simulink model "CLIK_Jpseudo_inv"  (R2023b)
settings: Solver=ode1  StartTime=0.0  StopTime=50  FixedStep=Tc  RelTol=1e-3
values from neighbouring files (symbols this model uses):
  Tc = 0.001    [scara_parameters.m]
undefined symbols (not defined in the file or in its folder): DiscIntNeverNeededParam, k0, K_Jpseudo_inv, q0
settings Model: Creator=emman  LastModifiedBy=emman

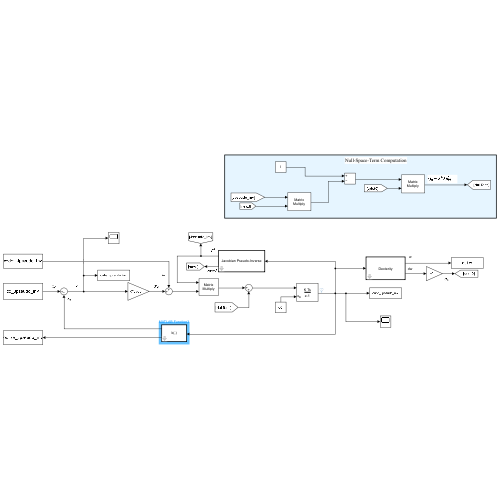
[thumbnail: Simulink's stored preview of the top-level diagram]
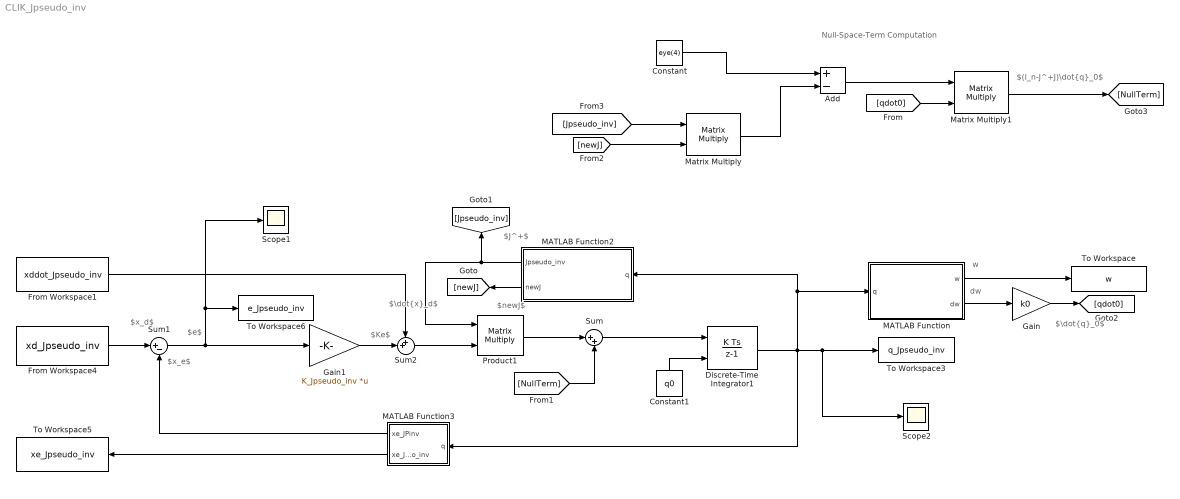
== system CLIK_Jpseudo_inv ==
  note: Null-Space-Term Computation
  note: $(I_n-J^+J)\dot{q}_0$
  note: $newJ$
  note: $J^+$
  note: $\dot{q}_0$
  note: dw
  note: w
  note: $Ke$
  note: $e$
  note: $\dot{x}_d$
  note: $x_d$
  note: $x_e$
  Add : Sum  Inputs=+-
  Constant : Constant  Value=eye(4)
      mask Display: disp('I');
  Constant1 : Constant  Value=q0
  Discrete-Time Integrator1 : DiscreteIntegrator  InitialConditionSource=external  InitialCondition=q0  SampleTime=Tc  ICPrevOutput=DiscIntNeverNeededParam  ICPrevScaledInput=DiscIntNeverNeededParam
  From Workspace1 : FromWorkspace  VariableName=xddot_Jpseudo_inv  SampleTime=Tc
  From Workspace4 : FromWorkspace  VariableName=xd_Jpseudo_inv  SampleTime=Tc
  Gain : Gain  Gain=k0
  Gain1 : Gain  Gain=K_Jpseudo_inv  Multiplication=Matrix(K*u) (u vector)
  MATLAB Function : MATLAB Function  TreatAsAtomicUnit=on
  MATLAB Function2 : MATLAB Function  TreatAsAtomicUnit=on
  MATLAB Function3 : MATLAB Function  TreatAsAtomicUnit=on
  Matrix Multiply : Product  Multiplication=Matrix(*)
  Matrix Multiply1 : Product  Multiplication=Matrix(*)
  Product1 : Product  Multiplication=Matrix(*)
  Scope1 : Scope
  Scope2 : Scope
  Sum : Sum  Inputs=|++
  Sum1 : Sum  Inputs=|+-
  Sum2 : Sum  Inputs=++|
  To Workspace : ToWorkspace  VariableName=w  SaveFormat=Structure With Time  SampleTime=-1
  To Workspace3 : ToWorkspace  VariableName=q_Jpseudo_inv  SaveFormat=Structure With Time  SampleTime=-1
  To Workspace5 : ToWorkspace  VariableName=xe_Jpseudo_inv  SaveFormat=Structure With Time  SampleTime=-1
  To Workspace6 : ToWorkspace  VariableName=e_Jpseudo_inv  SaveFormat=Structure With Time  SampleTime=-1
  wires:
  Discrete-Time Integrator1/1 -> MATLAB Function2/1(q), MATLAB Function/1(q), To Workspace3/1, Scope2/1, MATLAB Function3/1(q)
  From Workspace4/1 -> Sum1/1
  From Workspace1/1 -> Sum2/1
  Constant1/1 -> Discrete-Time Integrator1/2
  MATLAB Function2/1(Jpseudo_inv) -> Product1/1, [Jpseudo_inv]
  Gain1/1 -> Sum2/2
  Sum2/1 -> Product1/2
  Sum1/1 -> Scope1/1, To Workspace6/1, Gain1/1
  MATLAB Function/1(w) -> To Workspace/1
  MATLAB Function/2(dw) -> Gain/1
  MATLAB Function2/2(newJ) -> [newJ]
  Constant/1 -> Add/1
  [Jpseudo_inv] -> Matrix Multiply/1
  [newJ] -> Matrix Multiply/2
  Matrix Multiply/1 -> Add/2
  Gain/1 -> [qdot0]
  Add/1 -> Matrix Multiply1/1
  [qdot0] -> Matrix Multiply1/2
  Matrix Multiply1/1 -> [NullTerm]
  Product1/1 -> Sum/1
  Sum/1 -> Discrete-Time Integrator1/1
  [NullTerm] -> Sum/2
  MATLAB Function3/1(xe_JPinv) -> Sum1/2
  MATLAB Function3/2(xe_JPseudo_inv) -> To Workspace5/1

== matlab function CLIK_Jpseudo_inv/MATLAB Function2 ==
  data: Jpseudo_inv output; q input; newJ output
function [Jpseudo_inv,newJ] = JacobianPseudoInverse(q)

    a1 = 0.5;
    a2 = 0.5;
    
    newJ = [-a2*sin(q(1)+q(2))-a1*sin(q(1)) -a2*sin(q(1)+q(2)) 0 0;
        %a2*cos(q(1)+q(2))+a1*cos(q(1)) a2*cos(q(1)+q(2)) 0 0;
        0 0 -1 0;
        1 1 0 -1];

    Jpseudo_inv = newJ'*inv(newJ*newJ');

end

== matlab function CLIK_Jpseudo_inv/MATLAB Function3 ==
  data: xe_JPinv output; q input; xe_JPseudo_inv output
function [xe_JPinv, xe_JPseudo_inv] = DirKinPseudoInv(q)
    
    a1 = 0.5;
    a2 = 0.5;
    d0 = 1;
    
    xe_JPinv = [a2*cos(q(1)+q(2))+a1*cos(q(1));
       %a2*sin(q(1)+q(2))+a1*sin(q(1));
       d0-q(3);
       q(1)+q(2)-q(4)];

    xe_JPseudo_inv = [a2*cos(q(1)+q(2))+a1*cos(q(1));
       a2*sin(q(1)+q(2))+a1*sin(q(1));
       d0-q(3);
       q(1)+q(2)-q(4)];

end

== matlab function CLIK_Jpseudo_inv/MATLAB Function ==
  data: q input; w output; dw output
function [w,dw] = dexterity(q)

    w = (sin(q(2)))^2;  %Simplified Manipulability Measure
    wdot = 2*sin(q(2))*cos(q(2));   %Derivative of the Manipulability Measure
    dw = [0 wdot 0 0]';

end
